simulink model "synchronous_motorc"  (R2018a)
settings: Solver=ode4  StartTime=0.0  StopTime=inf  FixedStep=0.0001  RelTol=1e-3
InitFcn:
  | init_sync
values from neighbouring files (symbols this model uses):
  alpha_z = atan(R/X)    [init_syncc.m]
  I_f = 0.5    [init_syncc.m]
  L = declive/(2*50*pi)    (= 1.19366207319)    [Ex2_Task3A.m]    (also in init_syncc.m = 0.566144)
  M = 1.20765    [init_syncc.m]
  omega_e = f*2*pi    (= 314.159265359)    [init_syncc.m]
  R = 0    [init_syncc.m]
  Speed = 1500 * 2*pi/60    (= 157.079632679)    [init_syncc.m]
  U = U_rms * sqrt(2)    [init_syncc.m]
  U_rms = 220    [init_syncc.m]
  Z_mod = sqrt(X^2+R^2)    [init_syncc.m]
libraries: powerlib_meascontrol x2
settings Model: xpc_rtwmakecfg_data=_xpcnblib__xpcetherlib__xpcether8255xlib__xpcetherGbElib_  Creator=PedroVS  LastModifiedBy=Paula Cunha

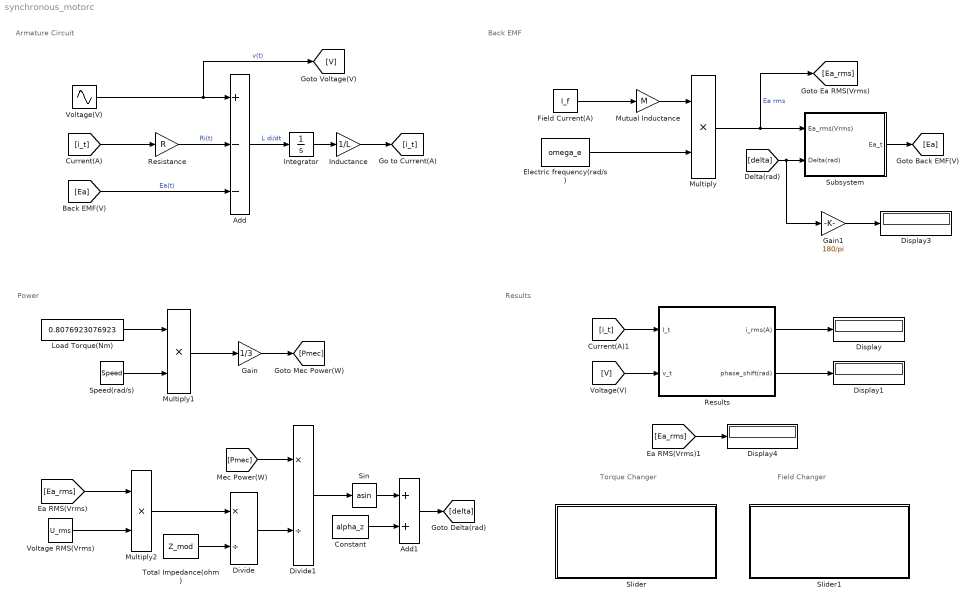
== system synchronous_motorc ==
  note: Torque Changer
  note: Results
  note: Power
  note: Back EMF
  note: Armature Circuit
  note: Field Changer
  Add : Sum  Inputs=+--
  Add1 : Sum
  Constant : Constant  Value=alpha_z
  Display{,1,3..4} (4 alike) : Display
  Divide : Product  Inputs=*/
  Divide1 : Product  Inputs=*/
  Electric frequency(rad/s) : Constant  Value=omega_e
  "Field Current(A) " : Constant  Value=I_f
  Gain : Gain  Gain=1/3
  Gain1 : Gain  Gain=180/pi
  Inductance : Gain  Gain=1/L
  Integrator : Integrator
  Load Torque(Nm) : Constant  Value=0.8076923076923
  Multiply : Product
  Multiply1 : Product
  Multiply2 : Product
  Mutual Inductance : Gain  Gain=M
  Resistance : Gain  Gain=R
  "Results " : Subsystem
  Sin : Trigonometry  Operator=asin
  Slider : Subsystem  DialogController=hmiCreateDDGDialog  IsWebBlock=on  mask(MWDashboardBlock){webBlockId=3a4f1ff3-74c4-4006-a939-74e4c5b97cdf, webBlockType=slider, ShowInLibBrowser=on, ShowInitialText=on, HMISrcModelName=synchronous_motor}
      mask prompts: webBlockId "WebBlock Id"; webBlockType "WebBlock Type"; HMISrcModelName "Source Model"
      mask help: SimulinkHMI:dialogs:SliderDialogDesc
      mask Help: helpview([docroot '/mapfiles/simulink.map'], 'hmi_slider')
      mask Display:
      | if strcmp(get_param(bdroot(gcb),'BlockDiagramType'), 'library')
      |     image([(matlabroot) '/toolbox/simulink/hmi/icons/Slider.png']);
      | end
  Slider1 : Subsystem  DialogController=hmiCreateDDGDialog  IsWebBlock=on  mask(MWDashboardBlock){webBlockId=1450d999-c629-4475-ab38-e2dbe4e4d37c, webBlockType=slider, ShowInLibBrowser=on, ShowInitialText=on, HMISrcModelName=synchronous_motor}
      mask prompts: webBlockId "WebBlock Id"; webBlockType "WebBlock Type"; HMISrcModelName "Source Model"
      mask help: SimulinkHMI:dialogs:SliderDialogDesc
      mask Help: helpview([docroot '/mapfiles/simulink.map'], 'hmi_slider')
      mask Display:
      | if strcmp(get_param(bdroot(gcb),'BlockDiagramType'), 'library')
      |     image([(matlabroot) '/toolbox/simulink/hmi/icons/Slider.png']);
      | end
  Speed(rad/s) : Constant  Value=Speed
  Subsystem : Subsystem
  Total Impedance(ohm) : Constant  Value=Z_mod
  Voltage RMS(Vrms) : Constant  Value=U_rms
  "Voltage(V) " : Sin  Amplitude=U  Frequency=omega_e  Phase=2*pi  SampleTime=0
  wires:
  Resistance/1 -> Add/2  "Ri(t)"
  [i_t] -> Resistance/1
  Add/1 -> Integrator/1  "L di/dt"
  Inductance/1 -> [i_t]
  Integrator/1 -> Inductance/1
  "Voltage(V) "/1 -> [V], Add/1  "v(t)"
  [Ea] -> Add/3  "Ea(t)"
  "Field Current(A) "/1 -> Mutual Inductance/1
  Mutual Inductance/1 -> Multiply/1
  Electric frequency(rad/s)/1 -> Multiply/2
  Multiply/1 -> [Ea_rms], Subsystem/1(Ea_rms(Vrms))  "Ea rms"
  Subsystem/1(Ea_t) -> [Ea]
  [delta] -> Gain1/1, Subsystem/2(Delta(rad))
  Load Torque(Nm)/1 -> Multiply1/1
  Speed(rad/s)/1 -> Multiply1/2
  Multiply1/1 -> Gain/1
  Gain/1 -> [Pmec]
  Voltage RMS(Vrms)/1 -> Multiply2/2
  [Ea_rms] -> Multiply2/1
  Multiply2/1 -> Divide/1
  Total Impedance(ohm)/1 -> Divide/2
  [Pmec] -> Divide1/1
  Divide1/1 -> Sin/1
  Sin/1 -> Add1/1
  Constant/1 -> Add1/2
  Add1/1 -> [delta]
  [i_t] -> "Results "/1(I_t)
  [V] -> "Results "/2("v_t ")
  "Results "/2(phase_shift(rad)) -> Display1/1
  "Results "/1("i_rms(A) ") -> Display/1
  Gain1/1 -> Display3/1
  [Ea_rms] -> Display4/1
  Divide/1 -> Divide1/2

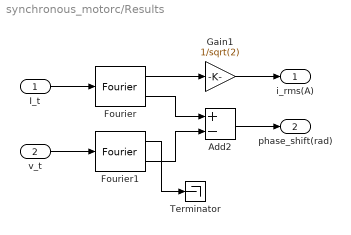
== system synchronous_motorc/Results  ==
  I_t : Inport
  "v_t " : Inport  Port=2
  Add2 : Sum  Inputs=+-
  Fourier : powerlib_meascontrol/Measurements/Fourier  Freq=50  n=1  InInit=[0, 0]  Ts=0
      settings: SourceProductName=Simscape Power Systems
  Fourier1 : powerlib_meascontrol/Measurements/Fourier  Freq=50  n=1  InInit=[0, 0]  Ts=0
      settings: SourceProductName=Simscape Power Systems
  Gain1 : Gain  Gain=1/sqrt(2)
  Terminator : Terminator
  "i_rms(A) " : Outport
  phase_shift(rad) : Outport  Port=2
  wires:
  Fourier1/2 -> Add2/2
  Fourier/2 -> Add2/1
  Fourier/1 -> Gain1/1
  I_t/1 -> Fourier/1
  "v_t "/1 -> Fourier1/1
  Gain1/1 -> "i_rms(A) "/1
  Add2/1 -> phase_shift(rad)/1
  Fourier1/1 -> Terminator/1

== system synchronous_motorc/Slider ==

== system synchronous_motorc/Slider1 ==

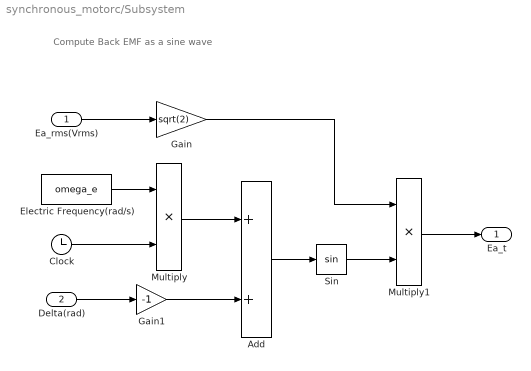
== system synchronous_motorc/Subsystem ==
  note: Compute Back EMF as a sine wave
  Ea_rms(Vrms) : Inport
  Delta(rad) : Inport  Port=2
  Add : Sum
  Clock : Clock
  Electric Frequency(rad/s) : Constant  Value=omega_e
  Gain : Gain  Gain=sqrt(2)
  Gain1 : Gain  Gain=-1
  Multiply : Product
  Multiply1 : Product
  Sin : Trigonometry
  Ea_t : Outport
  wires:
  Ea_rms(Vrms)/1 -> Gain/1
  Electric Frequency(rad/s)/1 -> Multiply/1
  Clock/1 -> Multiply/2
  Multiply/1 -> Add/1
  Delta(rad)/1 -> Gain1/1
  Add/1 -> Sin/1
  Gain/1 -> Multiply1/1
  Sin/1 -> Multiply1/2
  Multiply1/1 -> Ea_t/1
  Gain1/1 -> Add/2
